simulink model "Ecotron"  (R2019b)
settings: Solver=FixedStepAuto  StartTime=0.0  StopTime=1  FixedStep=0.001  RelTol=1e-3  EnableMultiTasking=on
InitFcn:
  | EcoCoder_PreCheckLic();
libraries: CoderSF_BSW_Libs x228, SF_CanService_Libs x49, simulink x33, dspstat3 x6
(part 5 of 6)

== system Ecotron/Input/PC/FrontWheelCommands/Subsystem1 ==
  "Available_in " : Inport
  Msg_cnt : Inport  Port=2
  Constant : Constant  Value=3  OutDataTypeStr=single
  Data Type Conversion : DataTypeConversion  OutDataTypeStr=single
  Delay1 : Delay  InitialCondition=0  SampleTime=0.5
  Delay2 : Delay  DelayLength=6  InitialCondition=0  SampleTime=0.5
  Delay3 : Delay  DelayLength=0  InitialCondition=0  SampleTime=0.5
  Divide : Product  Inputs=*/
  Relational Operator : RelationalOperator  Operator===  OutDataTypeStr=boolean  RndMeth=Simplest
  Subtract : Sum  Inputs=+-
  Write Measurement : CoderSF_BSW_Libs/Calibration & Measurement/Write Measurement  variable_name=PC_FrontwheelMsg_cnt  variable_value=0  variable_type=uint32  numD=1  unitStr=""  descStr=""
      settings: AttributesFormatString=type:%<variable_type> Dimensions:%<numD>  SourceProductName=EcoCoder Blocks
  Write Measurement1 : CoderSF_BSW_Libs/Calibration & Measurement/Write Measurement  variable_name=PC_FrontwheelMsg_Freq  variable_value=0  variable_type=single  numD=1  unitStr=""  descStr=""
      settings: AttributesFormatString=type:%<variable_type> Dimensions:%<numD>  SourceProductName=EcoCoder Blocks
  "Available " : Outport
  Cnt : Outport  Port=2
  Timeout_Err : Outport  Port=3
  Msg_Freq : Outport  Port=4
  wires:
  Delay3/1 -> Subtract/1
  Constant/1 -> Divide/2
  Divide/1 -> Write Measurement1/1, Msg_Freq/1
  Data Type Conversion/1 -> Divide/1
  Delay2/1 -> Subtract/2
  Delay1/1 -> Relational Operator/2
  Msg_cnt/1 -> Cnt/1, Delay2/1, Delay1/1, Write Measurement/1, Relational Operator/1, Delay3/1
  Relational Operator/1 -> Timeout_Err/1
  Subtract/1 -> Data Type Conversion/1
  "Available_in "/1 -> "Available "/1

== system Ecotron/Input/PC/LongitudinalCommands/Subsystem1 ==
  "Available_in " : Inport
  Msg_cnt : Inport  Port=2
  Constant : Constant  Value=3  OutDataTypeStr=single
  Data Type Conversion : DataTypeConversion  OutDataTypeStr=single
  Delay1 : Delay  InitialCondition=0  SampleTime=0.5
  Delay2 : Delay  DelayLength=6  InitialCondition=0  SampleTime=0.5
  Delay3 : Delay  DelayLength=0  InitialCondition=0  SampleTime=0.5
  Divide : Product  Inputs=*/
  Relational Operator : RelationalOperator  Operator===  OutDataTypeStr=boolean  RndMeth=Simplest
  Subtract : Sum  Inputs=+-
  "Available " : Outport
  Cnt : Outport  Port=2
  Timeout_Err : Outport  Port=3
  Msg_Freq : Outport  Port=4
  wires:
  "Available_in "/1 -> "Available "/1
  Subtract/1 -> Data Type Conversion/1
  Relational Operator/1 -> Timeout_Err/1
  Msg_cnt/1 -> Relational Operator/1, Delay3/1, Delay1/1, Delay2/1, Cnt/1
  Delay1/1 -> Relational Operator/2
  Delay2/1 -> Subtract/2
  Data Type Conversion/1 -> Divide/1
  Divide/1 -> Msg_Freq/1
  Constant/1 -> Divide/2
  Delay3/1 -> Subtract/1

== system Ecotron/Input/PC/LongitudinalCommandsV2/Subsystem1 ==
  "Available_in " : Inport
  Msg_cnt : Inport  Port=2
  Constant : Constant  Value=3  OutDataTypeStr=single
  Data Type Conversion : DataTypeConversion  OutDataTypeStr=single
  Delay1 : Delay  InitialCondition=0  SampleTime=0.5
  Delay2 : Delay  DelayLength=6  InitialCondition=0  SampleTime=0.5
  Delay3 : Delay  DelayLength=0  InitialCondition=0  SampleTime=0.5
  Divide : Product  Inputs=*/
  Relational Operator : RelationalOperator  Operator===  OutDataTypeStr=boolean  RndMeth=Simplest
  Subtract : Sum  Inputs=+-
  "Available " : Outport
  Cnt : Outport  Port=2
  Timeout_Err : Outport  Port=3
  Msg_Freq : Outport  Port=4
  wires:
  Delay3/1 -> Subtract/1
  Constant/1 -> Divide/2
  Divide/1 -> Msg_Freq/1
  Data Type Conversion/1 -> Divide/1
  Delay2/1 -> Subtract/2
  Delay1/1 -> Relational Operator/2
  Msg_cnt/1 -> Cnt/1, Delay2/1, Delay1/1, Delay3/1, Relational Operator/1
  Relational Operator/1 -> Timeout_Err/1
  Subtract/1 -> Data Type Conversion/1
  "Available_in "/1 -> "Available "/1

== system Ecotron/Input/PC/Vehicle_Commands/Subsystem1 ==
  "Available_in " : Inport
  Msg_cnt : Inport  Port=2
  Constant : Constant  Value=3  OutDataTypeStr=single
  Data Type Conversion : DataTypeConversion  OutDataTypeStr=single
  Delay1 : Delay  InitialCondition=0  SampleTime=0.5
  Delay2 : Delay  DelayLength=6  InitialCondition=0  SampleTime=0.5
  Delay3 : Delay  DelayLength=0  InitialCondition=0  SampleTime=0.5
  Divide : Product  Inputs=*/
  Relational Operator : RelationalOperator  Operator===  OutDataTypeStr=boolean  RndMeth=Simplest
  Subtract : Sum  Inputs=+-
  "Available " : Outport
  Cnt : Outport  Port=2
  Timeout_Err : Outport  Port=3
  Msg_Freq : Outport  Port=4
  wires:
  Delay3/1 -> Subtract/1
  Constant/1 -> Divide/2
  Divide/1 -> Msg_Freq/1
  Data Type Conversion/1 -> Divide/1
  Delay2/1 -> Subtract/2
  Delay1/1 -> Relational Operator/2
  Msg_cnt/1 -> Cnt/1, Delay2/1, Delay1/1, Delay3/1, Relational Operator/1
  Relational Operator/1 -> Timeout_Err/1
  Subtract/1 -> Data Type Conversion/1
  "Available_in "/1 -> "Available "/1

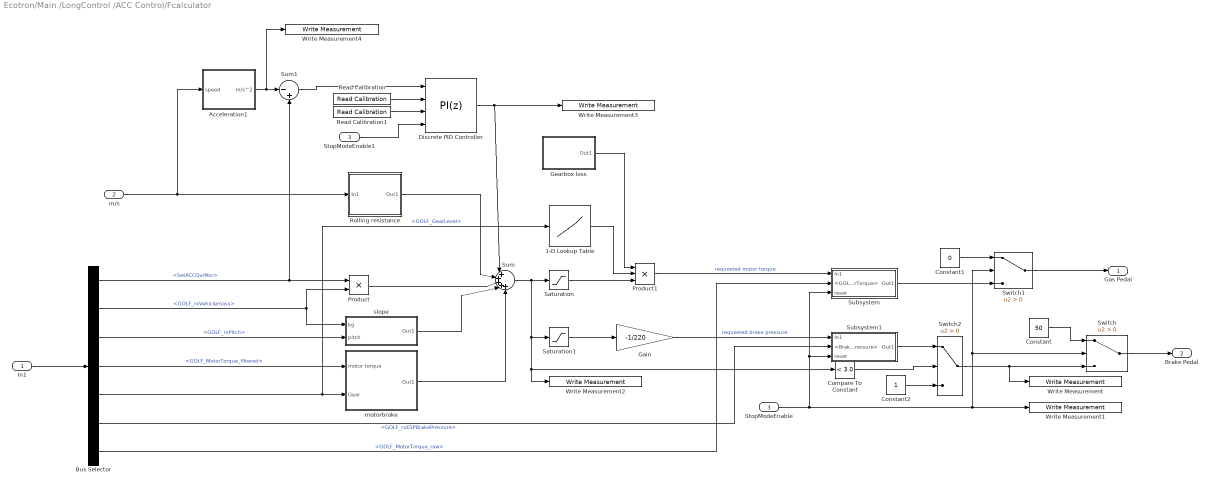
== system Ecotron/Main /LongControl /ACC Control/Fcalculator  ==
  In1 : Inport
  m/s : Inport  Port=2
  StopModeEnable : Inport  Port=3
  1-D Lookup Table : Lookup_n-D  NumberOfTableDimensions=1  BreakpointsForDimension1=[0 1 2 3 4 5]  Table=[0 1/53.5 1/32.6 1/21.7 1/16.2 1/12.2]  InternalRulePriority=Speed  RndMeth=Simplest  InputSameDT=on
  Acceleration1 : Subsystem
  Bus Selector : BusSelector  OutputSignals=input.PC.LongCMD.SetACCOvrMsr,input.vehicle.TSK.GOLF_rxVehiclemass,input.vehicle.TSK.GOLF_rxPitch,input.vehicle.MotorTorque.GOLF_MotorTorque_filtered,input.vehicle.GearLevel.GOLF_GearLevel,input.vehicle.BrakePressure.GOLF_rxESPBrakePressure,input.vehicle.MotorTorque.GOLF_MotorTorque_raw
  Compare To Constant : simulink/Logic and Bit Operations/Compare To Constant  relop=<  const=3.0  OutDataTypeStr=boolean
  Constant : Constant  Value=50  OutDataTypeStr=single
  Constant1 : Constant  Value=0  OutDataTypeStr=single
  Constant2 : Constant
  Discrete PID Controller : simulink/Continuous/PID Controller  Controller=PI  Form=Parallel  TimeDomain=Discrete-time  SampleTime=-1  IntegratorMethod=Forward Euler  FilterMethod=Forward Euler  ControllerParametersSource=external  P=1  I=1  D=0  UseFilter=off  N=100  TunerSelectOption=Transfer Function Based (PID Tuner App)  InitialConditionSource=internal  InitialConditionForIntegrator=0  InitialConditionForFilter=0  DifferentiatorICPrevScaledInput=0  ExternalReset=either  TrackingMode=off  Kt=1  LimitOutput=on  UpperSaturationLimit=300  LowerSaturationLimit=-300  LinearizeAsGain=off  AntiWindupMode=clamping  Kb=1  POutMin=[]  POutMax=[]  IOutMin=[]  IOutMax=[]  DOutMin=[]  DOutMax=[]  NOutMin=[]  NOutMax=[]  SumOutMin=[]  SumOutMax=[]  SaturationOutMin=[]  SaturationOutMax=[]  PParamMin=[]  PParamMax=[]  IParamMin=[]  IParamMax=[]  DParamMin=[]  DParamMax=[]  NParamMin=[]  NParamMax=[]  KbParamMin=[]  KbParamMax=[]  KtParamMin=[]  KtParamMax=[]  KbOutMin=[]  KbOutMax=[]  KtOutMin=[]  KtOutMax=[]  IntegratorOutMin=[]  IntegratorOutMax=[]  FilterOutMin=[]  FilterOutMax=[]  SumI1OutMin=[]  SumI1OutMax=[]  SumI2OutMin=[]  SumI2OutMax=[]  SumI3OutMin=[]  SumI3OutMax=[]  SumI4OutMin=[]  SumI4OutMax=[]  SumDOutMin=[]  SumDOutMax=[]  DifferentiatorOutMin=[]  DifferentiatorOutMax=[]  FilterDiffOutCoefMin=[]  FilterDiffOutCoefMax=[]  ReciprocalOutMin=[]  ReciprocalOutMax=[]  SumDenOutMin=[]  SumDenOutMax=[]  SumNumOutMin=[]  SumNumOutMax=[]  DivideOutMin=[]  DivideOutMax=[]  IntegratorContinuousStateAttributes=''  IntegratorStateMustResolveToSignalObject=off  IntegratorRTWStateStorageClass=Auto  FilterContinuousStateAttributes=''  FilterStateMustResolveToSignalObject=off  FilterRTWStateStorageClass=Auto  ParallelPVariant=ExternalParameters  IdealPVariant=Disabled  IVariant=ExternalParameters  DVariant=Disabled  IntegratorVariant=Discrete  SatVariant=Enabled  AWVariant=DiscClampingParallel  PCopyVariant=Disabled  TRVariant=Disabled  FdbkBlocksVariant=Forward  IdealPFdbkVariant=Disabled  SatFdbkVariant=Disabled  DerivativeFilterVariant=Disabled  NVariant=Disabled  NCopyVariant=Disabled_SignalSpec  FilterICVariant=Disabled  IntegratorICVariant=InternalICs  ExternalResetVariant=ExternalReset  TRSumVariant=Passthrough  SumFdbkVariant=Disabled  SumVariant=Sum_PI
  Gain : Gain  Gain=-1/220
  Gearbox loss : Subsystem
  Product : Product
  Product1 : Product  Inputs=3
  Read Calibration : CoderSF_BSW_Libs/Calibration & Measurement/Read Calibration  variable_name=Compensation_P  variable_value=300  variable_type=single  variable_min=[]  variable_max=[]  unitStr=""  descStr=""
      settings: AttributesFormatString=value:%<variable_value> type:%<variable_type> max:%<variable_max> Min:%<variable_min>
  Read Calibration1 : CoderSF_BSW_Libs/Calibration & Measurement/Read Calibration  variable_name=Compensation_I  variable_value=300  variable_type=single  variable_min=[]  variable_max=[]  unitStr=""  descStr=""
      settings: AttributesFormatString=value:%<variable_value> type:%<variable_type> max:%<variable_max> Min:%<variable_min>
  Rolling resistance : Subsystem
  Saturation : Saturate  UpperLimit=3000  LowerLimit=0
  Saturation1 : Saturate  UpperLimit=10  LowerLimit=-10000
  StopModeEnable1 : InportShadow  Port=3
  Subsystem : Subsystem
  Subsystem1 : Subsystem
  Sum : Sum  Inputs=|+++++
  Sum1 : Sum  Inputs=|-+
  Switch : Switch  Criteria=u2 > Threshold
  Switch1 : Switch  Criteria=u2 > Threshold
  Switch2 : Switch  Criteria=u2 > Threshold
  Write Measurement : CoderSF_BSW_Libs/Calibration & Measurement/Write Measurement  variable_name=debug_set_brake  variable_value=0  variable_type=single  numD=1  unitStr=""  descStr=""
      settings: AttributesFormatString=type:%<variable_type> Dimensions:%<numD>
  Write Measurement1 : CoderSF_BSW_Libs/Calibration & Measurement/Write Measurement  variable_name=debug_stopmode  variable_value=0  variable_type=boolean  numD=1  unitStr=""  descStr=""
      settings: AttributesFormatString=type:%<variable_type> Dimensions:%<numD>
  Write Measurement2 : CoderSF_BSW_Libs/Calibration & Measurement/Write Measurement  variable_name=debug_Fr_request  variable_value=0  variable_type=single  numD=1  unitStr=""  descStr=""
      settings: AttributesFormatString=type:%<variable_type> Dimensions:%<numD>
  Write Measurement3 : CoderSF_BSW_Libs/Calibration & Measurement/Write Measurement  variable_name=debug_CompensationPID_out  variable_value=0  variable_type=single  numD=1  unitStr=""  descStr=""
      settings: AttributesFormatString=type:%<variable_type> Dimensions:%<numD>
  Write Measurement4 : CoderSF_BSW_Libs/Calibration & Measurement/Write Measurement  variable_name=debug_filtered_ACC  variable_value=0  variable_type=single  numD=1  unitStr=""  descStr=""
      settings: AttributesFormatString=type:%<variable_type> Dimensions:%<numD>
  motorbrake : Subsystem
  slope : Subsystem
  Gas Pedal : Outport
  Brake Pedal : Outport  Port=2
  wires:
  In1/1 -> Bus Selector/1
  m/s/1 -> Acceleration1/1(speed), Rolling resistance/1(In1)
  Bus Selector/3 -> slope/2(pitch)  "<GOLF_rxPitch>"
  Bus Selector/2 -> slope/1(kg), Product/2  "<GOLF_rxVehiclemass>"
  Bus Selector/1 -> Sum1/2, Product/1  "<SetACCOvrMsr>"
  Bus Selector/4 -> motorbrake/1(motor torque)  "<GOLF_MotorTorque_filtered>"
  Bus Selector/5 -> motorbrake/2(Gear), 1-D Lookup Table/1  "<GOLF_GearLevel>"
  Rolling resistance/1(Out1) -> Sum/2
  Product/1 -> Sum/3
  slope/1(Out1) -> Sum/4
  motorbrake/1(Out1) -> Sum/5
  Sum/1 -> Write Measurement2/1, Compare To Constant/1, Saturation1/1, Saturation/1
  1-D Lookup Table/1 -> Product1/2
  Saturation/1 -> Product1/3
  Gearbox loss/1(Out1) -> Product1/1
  Saturation1/1 -> Gain/1
  Product1/1 -> Subsystem/1(In1)  "requested motor torque"
  Gain/1 -> Subsystem1/1(In1)  "requested brake pressure"
  Bus Selector/6 -> Subsystem1/2(<Brake pressure>)  "<GOLF_rxESPBrakePressure>"
  Constant1/1 -> Switch1/1
  Constant/1 -> Switch/1
  Subsystem/1(Out1) -> Switch1/3
  Switch1/1 -> Gas Pedal/1
  Switch2/1 -> Write Measurement/1, Switch/3
  Switch/1 -> Brake Pedal/1
  StopModeEnable/1 -> Subsystem/3(reset), Subsystem1/3(reset), Switch1/2, Switch/2, Write Measurement1/1
  Acceleration1/1(m/s^2) -> Write Measurement4/1, Sum1/1
  Sum1/1 -> Discrete PID Controller/1
  StopModeEnable1/1 -> Discrete PID Controller/4
  Read Calibration/1 -> Discrete PID Controller/2
  Read Calibration1/1 -> Discrete PID Controller/3
  Discrete PID Controller/1 -> Write Measurement3/1, Sum/1
  Bus Selector/7 -> Subsystem/2(<GOLF_MotorTorque>)  "<GOLF_MotorTorque_raw>"
  Subsystem1/1(Out1) -> Switch2/1
  Compare To Constant/1 -> Switch2/2
  Constant2/1 -> Switch2/3

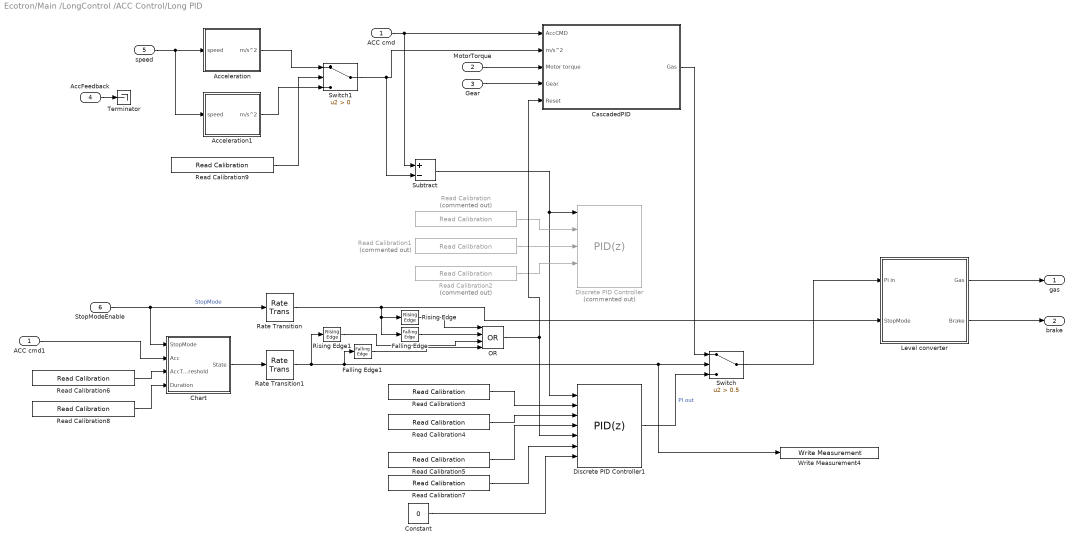
== system Ecotron/Main /LongControl /ACC Control/Long PID ==
  ACC cmd : Inport
  MotorTorque : Inport  Port=2
  Gear : Inport  Port=3
  AccFeedback : Inport  Port=4
  speed : Inport  Port=5
  StopModeEnable : Inport  Port=6
  ACC cmd1 : InportShadow
  Acceleration : Subsystem
  Acceleration1 : Subsystem
  CascadedPID : Subsystem
  Chart : Stateflow chart  BlockKeywords=__PRM__SERIALIZED__DATA__:Stateflow Chart,Stateflow Diagram  TreatAsAtomicUnit=on
  Constant : Constant  Value=0  OutDataTypeStr=single
  Discrete PID Controller : simulink/Continuous/PID Controller  Commented=on  Controller=PID  Form=Parallel  TimeDomain=Discrete-time  SampleTime=1/100  IntegratorMethod=Forward Euler  FilterMethod=Forward Euler  ControllerParametersSource=external  P=1  I=1  D=0  UseFilter=off  N=100  TunerSelectOption=Transfer Function Based (PID Tuner App)  ZeroCross=off  InitialConditionSource=internal  InitialConditionForIntegrator=0  InitialConditionForFilter=0  DifferentiatorICPrevScaledInput=0  ExternalReset=either  TrackingMode=off  Kt=1  LimitOutput=on  UpperSaturationLimit=0.5  LowerSaturationLimit=-0.1  LinearizeAsGain=off  AntiWindupMode=clamping  Kb=1  POutMin=[]  POutMax=[]  IOutMin=[]  IOutMax=[]  DOutMin=[]  DOutMax=[]  NOutMin=[]  NOutMax=[]  SumOutMin=[]  SumOutMax=[]  SaturationOutMin=[]  SaturationOutMax=[]  PParamMin=[]  PParamMax=[]  IParamMin=[]  IParamMax=[]  DParamMin=[]  DParamMax=[]  NParamMin=[]  NParamMax=[]  KbParamMin=[]  KbParamMax=[]  KtParamMin=[]  KtParamMax=[]  KbOutMin=[]  KbOutMax=[]  KtOutMin=[]  KtOutMax=[]  IntegratorOutMin=[]  IntegratorOutMax=[]  FilterOutMin=[]  FilterOutMax=[]  SumI1OutMin=[]  SumI1OutMax=[]  SumI2OutMin=[]  SumI2OutMax=[]  SumI3OutMin=[]  SumI3OutMax=[]  SumI4OutMin=[]  SumI4OutMax=[]  SumDOutMin=[]  SumDOutMax=[]  DifferentiatorOutMin=[]  DifferentiatorOutMax=[]  FilterDiffOutCoefMin=[]  FilterDiffOutCoefMax=[]  ReciprocalOutMin=[]  ReciprocalOutMax=[]  SumDenOutMin=[]  SumDenOutMax=[]  SumNumOutMin=[]  SumNumOutMax=[]  DivideOutMin=[]  DivideOutMax=[]  IntegratorContinuousStateAttributes=''  IntegratorStateMustResolveToSignalObject=off  IntegratorRTWStateStorageClass=Auto  FilterContinuousStateAttributes=''  FilterStateMustResolveToSignalObject=off  FilterRTWStateStorageClass=Auto  ParallelPVariant=ExternalParameters  IdealPVariant=Disabled  IVariant=ExternalParameters  DVariant=ExternalParameters  IntegratorVariant=Discrete  SatVariant=Enabled  AWVariant=DiscClampingParallel  PCopyVariant=Disabled  TRVariant=Disabled  FdbkBlocksVariant=Forward  IdealPFdbkVariant=Disabled  SatFdbkVariant=Disabled  DerivativeFilterVariant=Differentiator  NVariant=Passthrough  NCopyVariant=Disabled_SignalSpec  FilterICVariant=InternalICsDifferentiator  IntegratorICVariant=InternalICs  ExternalResetVariant=ExternalReset  TRSumVariant=Passthrough  SumFdbkVariant=Disabled  SumVariant=Sum_PID
  Discrete PID Controller1 : simulink/Continuous/PID Controller  Controller=PID  Form=Parallel  TimeDomain=Discrete-time  SampleTime=1/100  IntegratorMethod=Forward Euler  FilterMethod=Forward Euler  ControllerParametersSource=external  P=1  I=1  D=0  UseFilter=off  N=100  TunerSelectOption=Transfer Function Based (PID Tuner App)  ZeroCross=off  InitialConditionSource=external  InitialConditionForIntegrator=0  InitialConditionForFilter=0  DifferentiatorICPrevScaledInput=0  ExternalReset=either  TrackingMode=off  Kt=1  LimitOutput=on  UpperSaturationLimit=0.05  LowerSaturationLimit=-1  LinearizeAsGain=off  AntiWindupMode=clamping  Kb=1  POutMin=[]  POutMax=[]  IOutMin=[]  IOutMax=[]  DOutMin=[]  DOutMax=[]  NOutMin=[]  NOutMax=[]  SumOutMin=[]  SumOutMax=[]  SaturationOutMin=[]  SaturationOutMax=[]  PParamMin=[]  PParamMax=[]  IParamMin=[]  IParamMax=[]  DParamMin=[]  DParamMax=[]  NParamMin=[]  NParamMax=[]  KbParamMin=[]  KbParamMax=[]  KtParamMin=[]  KtParamMax=[]  KbOutMin=[]  KbOutMax=[]  KtOutMin=[]  KtOutMax=[]  IntegratorOutMin=[]  IntegratorOutMax=[]  FilterOutMin=[]  FilterOutMax=[]  SumI1OutMin=[]  SumI1OutMax=[]  SumI2OutMin=[]  SumI2OutMax=[]  SumI3OutMin=[]  SumI3OutMax=[]  SumI4OutMin=[]  SumI4OutMax=[]  SumDOutMin=[]  SumDOutMax=[]  DifferentiatorOutMin=[]  DifferentiatorOutMax=[]  FilterDiffOutCoefMin=[]  FilterDiffOutCoefMax=[]  ReciprocalOutMin=[]  ReciprocalOutMax=[]  SumDenOutMin=[]  SumDenOutMax=[]  SumNumOutMin=[]  SumNumOutMax=[]  DivideOutMin=[]  DivideOutMax=[]  IntegratorContinuousStateAttributes=''  IntegratorStateMustResolveToSignalObject=off  IntegratorRTWStateStorageClass=Auto  FilterContinuousStateAttributes=''  FilterStateMustResolveToSignalObject=off  FilterRTWStateStorageClass=Auto  ParallelPVariant=ExternalParameters  IdealPVariant=Disabled  IVariant=ExternalParameters  DVariant=ExternalParameters  IntegratorVariant=Discrete  SatVariant=Enabled  AWVariant=DiscClampingParallel  PCopyVariant=Disabled  TRVariant=Disabled  FdbkBlocksVariant=Forward  IdealPFdbkVariant=Disabled  SatFdbkVariant=Disabled  DerivativeFilterVariant=Differentiator  NVariant=Passthrough  NCopyVariant=Disabled_SignalSpec  FilterICVariant=ExternalICs  IntegratorICVariant=ExternalICs  ExternalResetVariant=ExternalReset  TRSumVariant=Passthrough  SumFdbkVariant=Disabled  SumVariant=Sum_PID
  Falling Edge : CoderSF_BSW_Libs/Application Base Blocks/Falling Edge  InitialCondition=off
      settings: SourceProductName=EcoCoder Blocks
  Falling Edge1 : CoderSF_BSW_Libs/Application Base Blocks/Falling Edge  InitialCondition=off
      settings: SourceProductName=EcoCoder Blocks
  Level converter : Subsystem
  OR : Logic  Operator=OR  Inputs=4  IconShape=distinctive  AllPortsSameDT=off  OutDataTypeStr=boolean
  Rate Transition : RateTransition  OutPortSampleTime=0.01
  Rate Transition1 : RateTransition  OutPortSampleTime=0.01
  Read Calibration : CoderSF_BSW_Libs/Calibration & Measurement/Read Calibration  Commented=on  variable_name=Acc_PID_P  variable_value=0.08  variable_type=single  variable_min=[]  variable_max=[]  unitStr=""  descStr=""
      settings: AttributesFormatString=value:%<variable_value> type:%<variable_type> max:%<variable_max> Min:%<variable_min>  SourceProductName=EcoCoder Blocks
  Read Calibration1 : CoderSF_BSW_Libs/Calibration & Measurement/Read Calibration  Commented=on  variable_name=Acc_PID_I  variable_value=0.15  variable_type=single  variable_min=[]  variable_max=[]  unitStr=""  descStr=""
      settings: AttributesFormatString=value:%<variable_value> type:%<variable_type> max:%<variable_max> Min:%<variable_min>  SourceProductName=EcoCoder Blocks
  Read Calibration2 : CoderSF_BSW_Libs/Calibration & Measurement/Read Calibration  Commented=on  variable_name=Acc_PID_D  variable_value=0.0  variable_type=single  variable_min=[]  variable_max=[]  unitStr=""  descStr=""
      settings: AttributesFormatString=value:%<variable_value> type:%<variable_type> max:%<variable_max> Min:%<variable_min>  SourceProductName=EcoCoder Blocks
  Read Calibration3 : CoderSF_BSW_Libs/Calibration & Measurement/Read Calibration  variable_name=Decc_PID_P  variable_value=0.05  variable_type=single  variable_min=[]  variable_max=[]  unitStr=""  descStr=""
      settings: AttributesFormatString=value:%<variable_value> type:%<variable_type> max:%<variable_max> Min:%<variable_min>  SourceProductName=EcoCoder Blocks
  Read Calibration4 : CoderSF_BSW_Libs/Calibration & Measurement/Read Calibration  variable_name=Decc_PID_I  variable_value=0.35  variable_type=single  variable_min=[]  variable_max=[]  unitStr=""  descStr=""
      settings: AttributesFormatString=value:%<variable_value> type:%<variable_type> max:%<variable_max> Min:%<variable_min>  SourceProductName=EcoCoder Blocks
  Read Calibration5 : CoderSF_BSW_Libs/Calibration & Measurement/Read Calibration  variable_name=Decc_PID_D  variable_value=0.0  variable_type=single  variable_min=[]  variable_max=[]  unitStr=""  descStr=""
      settings: AttributesFormatString=value:%<variable_value> type:%<variable_type> max:%<variable_max> Min:%<variable_min>  SourceProductName=EcoCoder Blocks
  Read Calibration6 : CoderSF_BSW_Libs/Calibration & Measurement/Read Calibration  variable_name=Acc_Threshold  variable_value=0.08  variable_type=single  variable_min=[]  variable_max=[]  unitStr=""  descStr=""
      settings: AttributesFormatString=value:%<variable_value> type:%<variable_type> max:%<variable_max> Min:%<variable_min>  SourceProductName=EcoCoder Blocks
  Read Calibration7 : CoderSF_BSW_Libs/Calibration & Measurement/Read Calibration  variable_name=Decc_PID_I0  variable_value=-0.05  variable_type=single  variable_min=[]  variable_max=[]  unitStr=""  descStr=""
      settings: AttributesFormatString=value:%<variable_value> type:%<variable_type> max:%<variable_max> Min:%<variable_min>  SourceProductName=EcoCoder Blocks
  Read Calibration8 : CoderSF_BSW_Libs/Calibration & Measurement/Read Calibration  variable_name=Acc_Duration  variable_value=0.8  variable_type=single  variable_min=[]  variable_max=[]  unitStr=""  descStr=""
      settings: AttributesFormatString=value:%<variable_value> type:%<variable_type> max:%<variable_max> Min:%<variable_min>  SourceProductName=EcoCoder Blocks
  Read Calibration9 : CoderSF_BSW_Libs/Calibration & Measurement/Read Calibration  variable_name=ACC_feedback  variable_value=0  variable_type=boolean  variable_min=[]  variable_max=[]  unitStr=bool  descStr="0 -> speed Derivative  1-> CAN"
      settings: AttributesFormatString=value:%<variable_value> type:%<variable_type> max:%<variable_max> Min:%<variable_min>  SourceProductName=EcoCoder Blocks
  Rising Edge : CoderSF_BSW_Libs/Application Base Blocks/Rising Edge  InitialCondition=on
      settings: SourceProductName=EcoCoder Blocks
  Rising Edge1 : CoderSF_BSW_Libs/Application Base Blocks/Rising Edge  InitialCondition=on
      settings: SourceProductName=EcoCoder Blocks
  Subtract : Sum  Inputs=+-
  Switch : Switch  Criteria=u2 > Threshold  Threshold=0.5
  Switch1 : Switch  Criteria=u2 > Threshold
  Terminator : Terminator
  Write Measurement4 : CoderSF_BSW_Libs/Calibration & Measurement/Write Measurement  variable_name=GasBrakeMode  variable_value=0  variable_type=boolean  numD=1  unitStr=""  descStr=""
      settings: AttributesFormatString=type:%<variable_type> Dimensions:%<numD>  SourceProductName=EcoCoder Blocks
  gas : Outport
  brake : Outport  Port=2
  wires:
  ACC cmd/1 -> CascadedPID/1(AccCMD), Subtract/1
  Subtract/1 -> Discrete PID Controller1/1, Discrete PID Controller/1
  Read Calibration/1 -> Discrete PID Controller/2
  Read Calibration1/1 -> Discrete PID Controller/3
  StopModeEnable/1 -> Chart/1(StopMode), Rate Transition/1  "StopMode"
  Level converter/2(Brake) -> brake/1
  Level converter/1(Gas) -> gas/1
  Read Calibration2/1 -> Discrete PID Controller/4
  Read Calibration3/1 -> Discrete PID Controller1/2
  Read Calibration4/1 -> Discrete PID Controller1/3
  Read Calibration5/1 -> Discrete PID Controller1/4
  Read Calibration6/1 -> Chart/3(AccThreshold)
  Chart/1(State) -> Rate Transition1/1
  Discrete PID Controller1/1 -> Switch/3  "PI out"
  Switch/1 -> Level converter/1(Pi in)
  OR/1 -> CascadedPID/5("Reset "), Discrete PID Controller1/5
  Constant/1 -> Discrete PID Controller1/7
  Read Calibration7/1 -> Discrete PID Controller1/6
  Rising Edge/1 -> OR/1
  Falling Edge/1 -> OR/2
  Rising Edge1/1 -> OR/3
  Falling Edge1/1 -> OR/4
  Rate Transition/1 -> Falling Edge/1, Rising Edge/1, Level converter/2(StopMode)
  Rate Transition1/1 -> Falling Edge1/1, Write Measurement4/1, Switch/2, Rising Edge1/1
  speed/1 -> Acceleration1/1(speed), Acceleration/1(speed)
  MotorTorque/1 -> CascadedPID/3(Motor torque)
  Gear/1 -> CascadedPID/4(Gear)
  CascadedPID/1(Gas) -> Switch/1
  Read Calibration8/1 -> Chart/4(Duration)
  Acceleration/1(m/s^2) -> Switch1/1
  Switch1/1 -> Subtract/2, CascadedPID/2(m/s^2)
  Read Calibration9/1 -> Switch1/2
  AccFeedback/1 -> Terminator/1
  Acceleration1/1(m/s^2) -> Switch1/3
  ACC cmd1/1 -> Chart/2(Acc)

== system Ecotron/Main /LongControl /ACC Control/StopModeDesicion ==
  note: 1 P
      | 2 R
      | 3 N
      | 4 D
  speed : Inport
  bus : Inport  Port=2
  Bus Selector : BusSelector  OutputSignals=input.PC.LongCMD.SetACCOvrMsr,input.vehicle.gear.GOLF_CurrentGear,mode
  Chart1 : Stateflow chart  BlockKeywords=__PRM__SERIALIZED__DATA__:Stateflow Chart,Stateflow Diagram  TreatAsAtomicUnit=on
  StopModeEnable : Outport
  wires:
  bus/1 -> Bus Selector/1
  speed/1 -> Chart1/4(Speed)
  Bus Selector/2 -> Chart1/2(Gear)  "<GOLF_CurrentGear>"
  Bus Selector/1 -> Chart1/1(Acc)  "<SetACCOvrMsr>"
  Chart1/1(Stopmode) -> StopModeEnable/1
  Bus Selector/3 -> Chart1/3(mode)  "<mode>"

== system Ecotron/Main /LongControl /ACC Control/VehicleSpeed ==
  In1 : Inport
  Bus Selector : BusSelector  OutputSignals=input.vehicle.WheelSpeed.GOLF_BLWheelSpeed,input.vehicle.WheelSpeed.GOLF_BRWheelSpeed
  Multiply : Gain  Gain=0.5
  Multiply1 : Gain  Gain=1/3.6
  Sum : Sum  Inputs=|++
  m/s : Outport
  wires:
  In1/1 -> Bus Selector/1
  Bus Selector/1 -> Sum/1  "<GOLF_BLWheelSpeed>"
  Bus Selector/2 -> Sum/2  "<GOLF_BRWheelSpeed>"
  Sum/1 -> Multiply/1
  Multiply/1 -> Multiply1/1
  Multiply1/1 -> m/s/1

== system Ecotron/Input/By-wire/PDS/Subsystem/Subsystem4 ==
  "Available_in " : Inport
  Msg_cnt : Inport  Port=2
  Constant : Constant  Value=3  OutDataTypeStr=single
  Data Type Conversion : DataTypeConversion  OutDataTypeStr=single
  Delay1 : Delay  InitialCondition=0  SampleTime=0.5
  Delay2 : Delay  DelayLength=6  InitialCondition=0  SampleTime=0.5
  Delay3 : Delay  DelayLength=0  InitialCondition=0  SampleTime=0.5
  Divide : Product  Inputs=*/
  Relational Operator : RelationalOperator  Operator===  OutDataTypeStr=boolean  RndMeth=Simplest
  Subtract : Sum  Inputs=+-
  "Available " : Outport
  Cnt : Outport  Port=2
  Timeout_Err : Outport  Port=3
  Msg_Freq : Outport  Port=4
  wires:
  "Available_in "/1 -> "Available "/1
  Subtract/1 -> Data Type Conversion/1
  Relational Operator/1 -> Timeout_Err/1
  Msg_cnt/1 -> Relational Operator/1, Delay3/1, Delay1/1, Delay2/1, Cnt/1
  Delay1/1 -> Relational Operator/2
  Delay2/1 -> Subtract/2
  Data Type Conversion/1 -> Divide/1
  Divide/1 -> Msg_Freq/1
  Constant/1 -> Divide/2
  Delay3/1 -> Subtract/1

== system Ecotron/Input/By-wire/PDS/Subsystem1/Subsystem6 ==
  "Available_in " : Inport
  Msg_cnt : Inport  Port=2
  Constant : Constant  Value=3  OutDataTypeStr=single
  Data Type Conversion : DataTypeConversion  OutDataTypeStr=single
  Delay1 : Delay  InitialCondition=0  SampleTime=0.5
  Delay2 : Delay  DelayLength=6  InitialCondition=0  SampleTime=0.5
  Delay3 : Delay  DelayLength=0  InitialCondition=0  SampleTime=0.5
  Divide : Product  Inputs=*/
  Relational Operator : RelationalOperator  Operator===  OutDataTypeStr=boolean  RndMeth=Simplest
  Subtract : Sum  Inputs=+-
  "Available " : Outport
  Cnt : Outport  Port=2
  Timeout_Err : Outport  Port=3
  Msg_Freq : Outport  Port=4
  wires:
  "Available_in "/1 -> "Available "/1
  Subtract/1 -> Data Type Conversion/1
  Relational Operator/1 -> Timeout_Err/1
  Msg_cnt/1 -> Relational Operator/1, Delay3/1, Delay1/1, Delay2/1, Cnt/1
  Delay1/1 -> Relational Operator/2
  Delay2/1 -> Subtract/2
  Data Type Conversion/1 -> Divide/1
  Divide/1 -> Msg_Freq/1
  Constant/1 -> Divide/2
  Delay3/1 -> Subtract/1

== system Ecotron/Input/By-wire/PDS/Subsystem2/Subsystem1 ==
  "Available_in " : Inport
  Msg_cnt : Inport  Port=2
  Constant : Constant  Value=3  OutDataTypeStr=single
  Data Type Conversion : DataTypeConversion  OutDataTypeStr=single
  Delay1 : Delay  InitialCondition=0  SampleTime=0.5
  Delay2 : Delay  DelayLength=6  InitialCondition=0  SampleTime=0.5
  Delay3 : Delay  DelayLength=0  InitialCondition=0  SampleTime=0.5
  Divide : Product  Inputs=*/
  Relational Operator : RelationalOperator  Operator===  OutDataTypeStr=boolean  RndMeth=Simplest
  Subtract : Sum  Inputs=+-
  "Available " : Outport
  Cnt : Outport  Port=2
  Timeout_Err : Outport  Port=3
  Msg_Freq : Outport  Port=4
  wires:
  "Available_in "/1 -> "Available "/1
  Subtract/1 -> Data Type Conversion/1
  Relational Operator/1 -> Timeout_Err/1
  Msg_cnt/1 -> Relational Operator/1, Delay3/1, Delay1/1, Delay2/1, Cnt/1
  Delay1/1 -> Relational Operator/2
  Delay2/1 -> Subtract/2
  Data Type Conversion/1 -> Divide/1
  Divide/1 -> Msg_Freq/1
  Constant/1 -> Divide/2
  Delay3/1 -> Subtract/1

== system Ecotron/Input/By-wire/PDS/Subsystem3/Subsystem2 ==
  "Available_in " : Inport
  Msg_cnt : Inport  Port=2
  Constant : Constant  Value=3  OutDataTypeStr=single
  Data Type Conversion : DataTypeConversion  OutDataTypeStr=single
  Delay1 : Delay  InitialCondition=0  SampleTime=0.5
  Delay2 : Delay  DelayLength=6  InitialCondition=0  SampleTime=0.5
  Delay3 : Delay  DelayLength=0  InitialCondition=0  SampleTime=0.5
  Divide : Product  Inputs=*/
  Relational Operator : RelationalOperator  Operator===  OutDataTypeStr=boolean  RndMeth=Simplest
  Subtract : Sum  Inputs=+-
  "Available " : Outport
  Cnt : Outport  Port=2
  Timeout_Err : Outport  Port=3
  Msg_Freq : Outport  Port=4
  wires:
  "Available_in "/1 -> "Available "/1
  Subtract/1 -> Data Type Conversion/1
  Relational Operator/1 -> Timeout_Err/1
  Msg_cnt/1 -> Relational Operator/1, Delay3/1, Delay1/1, Delay2/1, Cnt/1
  Delay1/1 -> Relational Operator/2
  Delay2/1 -> Subtract/2
  Data Type Conversion/1 -> Divide/1
  Divide/1 -> Msg_Freq/1
  Constant/1 -> Divide/2
  Delay3/1 -> Subtract/1

== system Ecotron/Input/By-wire/PDS/Subsystem4/Subsystem3 ==
  "Available_in " : Inport
  Msg_cnt : Inport  Port=2
  Constant : Constant  Value=3  OutDataTypeStr=single
  Data Type Conversion : DataTypeConversion  OutDataTypeStr=single
  Delay1 : Delay  InitialCondition=0  SampleTime=0.5
  Delay2 : Delay  DelayLength=6  InitialCondition=0  SampleTime=0.5
  Delay3 : Delay  DelayLength=0  InitialCondition=0  SampleTime=0.5
  Divide : Product  Inputs=*/
  Relational Operator : RelationalOperator  Operator===  OutDataTypeStr=boolean  RndMeth=Simplest
  Subtract : Sum  Inputs=+-
  "Available " : Outport
  Cnt : Outport  Port=2
  Timeout_Err : Outport  Port=3
  Msg_Freq : Outport  Port=4
  wires:
  "Available_in "/1 -> "Available "/1
  Subtract/1 -> Data Type Conversion/1
  Relational Operator/1 -> Timeout_Err/1
  Msg_cnt/1 -> Relational Operator/1, Delay3/1, Delay1/1, Delay2/1, Cnt/1
  Delay1/1 -> Relational Operator/2
  Delay2/1 -> Subtract/2
  Data Type Conversion/1 -> Divide/1
  Divide/1 -> Msg_Freq/1
  Constant/1 -> Divide/2
  Delay3/1 -> Subtract/1

== system Ecotron/Input/By-wire/PDS/Subsystem6/Subsystem5 ==
  "Available_in " : Inport
  Msg_cnt : Inport  Port=2
  Constant : Constant  Value=3  OutDataTypeStr=single
  Data Type Conversion : DataTypeConversion  OutDataTypeStr=single
  Delay1 : Delay  InitialCondition=0  SampleTime=0.5
  Delay2 : Delay  DelayLength=6  InitialCondition=0  SampleTime=0.5
  Delay3 : Delay  DelayLength=0  InitialCondition=0  SampleTime=0.5
  Divide : Product  Inputs=*/
  Relational Operator : RelationalOperator  Operator===  OutDataTypeStr=boolean  RndMeth=Simplest
  Subtract : Sum  Inputs=+-
  "Available " : Outport
  Cnt : Outport  Port=2
  Timeout_Err : Outport  Port=3
  Msg_Freq : Outport  Port=4
  wires:
  "Available_in "/1 -> "Available "/1
  Subtract/1 -> Data Type Conversion/1
  Relational Operator/1 -> Timeout_Err/1
  Msg_cnt/1 -> Relational Operator/1, Delay3/1, Delay1/1, Delay2/1, Cnt/1
  Delay1/1 -> Relational Operator/2
  Delay2/1 -> Subtract/2
  Data Type Conversion/1 -> Divide/1
  Divide/1 -> Msg_Freq/1
  Constant/1 -> Divide/2
  Delay3/1 -> Subtract/1

== system Ecotron/Input/By-wire/Robeff Brake ECU/Robeff Brake FbMsg1/Subsystem4 ==
  "Available_in " : Inport
  Msg_cnt : Inport  Port=2
  Constant : Constant  Value=3  OutDataTypeStr=single
  Data Type Conversion : DataTypeConversion  OutDataTypeStr=single
  Delay1 : Delay  InitialCondition=0  SampleTime=0.5
  Delay2 : Delay  DelayLength=6  InitialCondition=0  SampleTime=0.5
  Delay3 : Delay  DelayLength=0  InitialCondition=0  SampleTime=0.5
  Divide : Product  Inputs=*/
  Relational Operator : RelationalOperator  Operator===  OutDataTypeStr=boolean  RndMeth=Simplest
  Subtract : Sum  Inputs=+-
  "Available " : Outport
  Cnt : Outport  Port=2
  Timeout_Err : Outport  Port=3
  Msg_Freq : Outport  Port=4
  wires:
  Delay3/1 -> Subtract/1
  Constant/1 -> Divide/2
  Divide/1 -> Msg_Freq/1
  Data Type Conversion/1 -> Divide/1
  Delay2/1 -> Subtract/2
  Delay1/1 -> Relational Operator/2
  Msg_cnt/1 -> Cnt/1, Delay2/1, Delay1/1, Delay3/1, Relational Operator/1
  Relational Operator/1 -> Timeout_Err/1
  Subtract/1 -> Data Type Conversion/1
  "Available_in "/1 -> "Available "/1

== system Ecotron/Input/By-wire/Robeff Brake ECU/Robeff Brake FbMsg2/Subsystem4 ==
  "Available_in " : Inport
  Msg_cnt : Inport  Port=2
  Constant : Constant  Value=3  OutDataTypeStr=single
  Data Type Conversion : DataTypeConversion  OutDataTypeStr=single
  Delay1 : Delay  InitialCondition=0  SampleTime=0.5
  Delay2 : Delay  DelayLength=6  InitialCondition=0  SampleTime=0.5
  Delay3 : Delay  DelayLength=0  InitialCondition=0  SampleTime=0.5
  Divide : Product  Inputs=*/
  Relational Operator : RelationalOperator  Operator===  OutDataTypeStr=boolean  RndMeth=Simplest
  Subtract : Sum  Inputs=+-
  "Available " : Outport
  Cnt : Outport  Port=2
  Timeout_Err : Outport  Port=3
  Msg_Freq : Outport  Port=4
  wires:
  Delay3/1 -> Subtract/1
  Constant/1 -> Divide/2
  Divide/1 -> Msg_Freq/1
  Data Type Conversion/1 -> Divide/1
  Delay2/1 -> Subtract/2
  Delay1/1 -> Relational Operator/2
  Msg_cnt/1 -> Cnt/1, Delay2/1, Delay1/1, Delay3/1, Relational Operator/1
  Relational Operator/1 -> Timeout_Err/1
  Subtract/1 -> Data Type Conversion/1
  "Available_in "/1 -> "Available "/1

== system Ecotron/Input/By-wire/Robeff Brake ECU/Robeff Brake FbMsg3/Subsystem4 ==
  "Available_in " : Inport
  Msg_cnt : Inport  Port=2
  Constant : Constant  Value=3  OutDataTypeStr=single
  Data Type Conversion : DataTypeConversion  OutDataTypeStr=single
  Delay1 : Delay  InitialCondition=0  SampleTime=0.5
  Delay2 : Delay  DelayLength=6  InitialCondition=0  SampleTime=0.5
  Delay3 : Delay  DelayLength=0  InitialCondition=0  SampleTime=0.5
  Divide : Product  Inputs=*/
  Relational Operator : RelationalOperator  Operator===  OutDataTypeStr=boolean  RndMeth=Simplest
  Subtract : Sum  Inputs=+-
  "Available " : Outport
  Cnt : Outport  Port=2
  Timeout_Err : Outport  Port=3
  Msg_Freq : Outport  Port=4
  wires:
  Delay3/1 -> Subtract/1
  Constant/1 -> Divide/2
  Divide/1 -> Msg_Freq/1
  Data Type Conversion/1 -> Divide/1
  Delay2/1 -> Subtract/2
  Delay1/1 -> Relational Operator/2
  Msg_cnt/1 -> Cnt/1, Delay2/1, Delay1/1, Delay3/1, Relational Operator/1
  Relational Operator/1 -> Timeout_Err/1
  Subtract/1 -> Data Type Conversion/1
  "Available_in "/1 -> "Available "/1

== system Ecotron/Input/By-wire/Robeff EPAS ECU/Robeff EPAS FbMsg1/Subsystem4 ==
  "Available_in " : Inport
  Msg_cnt : Inport  Port=2
  Constant : Constant  Value=3
  Data Type Conversion : DataTypeConversion  OutDataTypeStr=single
  Delay1 : Delay  InitialCondition=0  SampleTime=0.5
  Delay2 : Delay  DelayLength=6  InitialCondition=0  SampleTime=0.5
  Delay3 : Delay  DelayLength=0  InitialCondition=0  SampleTime=0.5
  Divide : Product  Inputs=*/  OutDataTypeStr=single
  Relational Operator : RelationalOperator  Operator===  OutDataTypeStr=boolean  RndMeth=Simplest
  Subtract : Sum  Inputs=+-
  "Available " : Outport
  Cnt : Outport  Port=2
  Timeout_Err : Outport  Port=3
  Msg_Freq : Outport  Port=4
  wires:
  "Available_in "/1 -> "Available "/1
  Subtract/1 -> Data Type Conversion/1
  Relational Operator/1 -> Timeout_Err/1
  Msg_cnt/1 -> Relational Operator/1, Delay3/1, Delay1/1, Delay2/1, Cnt/1
  Delay1/1 -> Relational Operator/2
  Delay2/1 -> Subtract/2
  Data Type Conversion/1 -> Divide/1
  Divide/1 -> Msg_Freq/1
  Constant/1 -> Divide/2
  Delay3/1 -> Subtract/1

== system Ecotron/Input/By-wire/Robeff EPAS ECU/Robeff EPAS FbMsg2/Subsystem4 ==
  "Available_in " : Inport
  Msg_cnt : Inport  Port=2
  Constant : Constant  Value=3
  Data Type Conversion : DataTypeConversion  OutDataTypeStr=single
  Delay1 : Delay  InitialCondition=0  SampleTime=0.5
  Delay2 : Delay  DelayLength=6  InitialCondition=0  SampleTime=0.5
  Delay3 : Delay  DelayLength=0  InitialCondition=0  SampleTime=0.5
  Divide : Product  Inputs=*/  OutDataTypeStr=single
  Relational Operator : RelationalOperator  Operator===  OutDataTypeStr=boolean  RndMeth=Simplest
  Subtract : Sum  Inputs=+-
  "Available " : Outport
  Cnt : Outport  Port=2
  Timeout_Err : Outport  Port=3
  Msg_Freq : Outport  Port=4
  wires:
  "Available_in "/1 -> "Available "/1
  Subtract/1 -> Data Type Conversion/1
  Relational Operator/1 -> Timeout_Err/1
  Msg_cnt/1 -> Relational Operator/1, Delay3/1, Delay1/1, Delay2/1, Cnt/1
  Delay1/1 -> Relational Operator/2
  Delay2/1 -> Subtract/2
  Data Type Conversion/1 -> Divide/1
  Divide/1 -> Msg_Freq/1
  Constant/1 -> Divide/2
  Delay3/1 -> Subtract/1

== system Ecotron/Input/By-wire/Robeff EPAS ECU/Robeff EPAS FbMsg3/Subsystem4 ==
  "Available_in " : Inport
  Msg_cnt : Inport  Port=2
  Constant : Constant  Value=3
  Data Type Conversion : DataTypeConversion  OutDataTypeStr=single
  Delay1 : Delay  InitialCondition=0  SampleTime=0.5
  Delay2 : Delay  DelayLength=6  InitialCondition=0  SampleTime=0.5
  Delay3 : Delay  DelayLength=0  InitialCondition=0  SampleTime=0.5
  Divide : Product  Inputs=*/  OutDataTypeStr=single
  Relational Operator : RelationalOperator  Operator===  OutDataTypeStr=boolean  RndMeth=Simplest
  Subtract : Sum  Inputs=+-
  "Available " : Outport
  Cnt : Outport  Port=2
  Timeout_Err : Outport  Port=3
  Msg_Freq : Outport  Port=4
  wires:
  "Available_in "/1 -> "Available "/1
  Subtract/1 -> Data Type Conversion/1
  Relational Operator/1 -> Timeout_Err/1
  Msg_cnt/1 -> Relational Operator/1, Delay3/1, Delay1/1, Delay2/1, Cnt/1
  Delay1/1 -> Relational Operator/2
  Delay2/1 -> Subtract/2
  Data Type Conversion/1 -> Divide/1
  Divide/1 -> Msg_Freq/1
  Constant/1 -> Divide/2
  Delay3/1 -> Subtract/1

== system Ecotron/Main /LongControl /ACC Control/Fcalculator /Acceleration1 ==
  speed : Inport
  Moving Average1 : dspstat3/Moving Average  Method=Sliding window  ForgettingFactorPort=off  SpecifyWindowLength=on  WindowLength=200  ForgettingFactor=0.9  SimulateUsing=Code generation
  Moving Average2 : dspstat3/Moving Average  Method=Sliding window  ForgettingFactorPort=off  SpecifyWindowLength=on  WindowLength=200  ForgettingFactor=0.9  SimulateUsing=Code generation
  basic derivative1 : Subsystem
  m/s^2 : Outport
  wires:
  Moving Average2/1 -> m/s^2/1  "m/s^2"
  basic derivative1/1(Out1) -> Moving Average2/1
  speed/1 -> Moving Average1/1
  Moving Average1/1 -> basic derivative1/1(In1)  "m/s"

== system Ecotron/Main /LongControl /ACC Control/Fcalculator /Gearbox loss ==
  Constant : Constant  Value=1.06
  Out1 : Outport
  wires:
  Constant/1 -> Out1/1

== system Ecotron/Main /LongControl /ACC Control/Fcalculator /Rolling resistance ==
  In1 : Inport
  1-D Lookup Table : Lookup_n-D  NumberOfTableDimensions=1  BreakpointsForDimension1=[0 0.02 8 16]  Table=[0 163.2 228.5 326.4]  InternalRulePriority=Speed  RndMeth=Simplest  InputSameDT=on
  Out1 : Outport
  wires:
  1-D Lookup Table/1 -> Out1/1
  In1/1 -> 1-D Lookup Table/1

== system Ecotron/Main /LongControl /ACC Control/Fcalculator /Subsystem ==
  In1 : Inport
  <GOLF_MotorTorque> : Inport  Port=2
  reset : Inport  Port=3
  PID Controller1 : simulink/Continuous/PID Controller  Controller=PID  Form=Parallel  TimeDomain=Discrete-time  SampleTime=1/100  IntegratorMethod=Forward Euler  FilterMethod=Forward Euler  ControllerParametersSource=external  P=1  I=1  D=0  UseFilter=off  N=100  TunerSelectOption=Transfer Function Based (PID Tuner App)  ZeroCross=off  InitialConditionSource=internal  InitialConditionForIntegrator=0  InitialConditionForFilter=0  DifferentiatorICPrevScaledInput=0  ExternalReset=either  TrackingMode=off  Kt=1  LimitOutput=on  UpperSaturationLimit=50  LowerSaturationLimit=0  LinearizeAsGain=off  AntiWindupMode=clamping  Kb=1  POutMin=[]  POutMax=[]  IOutMin=[]  IOutMax=[]  DOutMin=[]  DOutMax=[]  NOutMin=[]  NOutMax=[]  SumOutMin=[]  SumOutMax=[]  SaturationOutMin=[]  SaturationOutMax=[]  PParamMin=[]  PParamMax=[]  IParamMin=[]  IParamMax=[]  DParamMin=[]  DParamMax=[]  NParamMin=[]  NParamMax=[]  KbParamMin=[]  KbParamMax=[]  KtParamMin=[]  KtParamMax=[]  KbOutMin=[]  KbOutMax=[]  KtOutMin=[]  KtOutMax=[]  IntegratorOutMin=[]  IntegratorOutMax=[]  FilterOutMin=[]  FilterOutMax=[]  SumI1OutMin=[]  SumI1OutMax=[]  SumI2OutMin=[]  SumI2OutMax=[]  SumI3OutMin=[]  SumI3OutMax=[]  SumI4OutMin=[]  SumI4OutMax=[]  SumDOutMin=[]  SumDOutMax=[]  DifferentiatorOutMin=[]  DifferentiatorOutMax=[]  FilterDiffOutCoefMin=[]  FilterDiffOutCoefMax=[]  ReciprocalOutMin=[]  ReciprocalOutMax=[]  SumDenOutMin=[]  SumDenOutMax=[]  SumNumOutMin=[]  SumNumOutMax=[]  DivideOutMin=[]  DivideOutMax=[]  IntegratorContinuousStateAttributes=''  IntegratorStateMustResolveToSignalObject=off  IntegratorRTWStateStorageClass=Auto  FilterContinuousStateAttributes=''  FilterStateMustResolveToSignalObject=off  FilterRTWStateStorageClass=Auto  ParallelPVariant=ExternalParameters  IdealPVariant=Disabled  IVariant=ExternalParameters  DVariant=ExternalParameters  IntegratorVariant=Discrete  SatVariant=Enabled  AWVariant=DiscClampingParallel  PCopyVariant=Disabled  TRVariant=Disabled  FdbkBlocksVariant=Forward  IdealPFdbkVariant=Disabled  SatFdbkVariant=Disabled  DerivativeFilterVariant=Differentiator  NVariant=Passthrough  NCopyVariant=Disabled_SignalSpec  FilterICVariant=InternalICsDifferentiator  IntegratorICVariant=InternalICs  ExternalResetVariant=ExternalReset  TRSumVariant=Passthrough  SumFdbkVariant=Disabled  SumVariant=Sum_PID
  Read Calibration : CoderSF_BSW_Libs/Calibration & Measurement/Read Calibration  variable_name=Torque_PID_P  variable_value=0.05  variable_type=single  variable_min=[]  variable_max=[]  unitStr=""  descStr=""
      settings: AttributesFormatString=value:%<variable_value> type:%<variable_type> max:%<variable_max> Min:%<variable_min>  SourceProductName=EcoCoder Blocks
  Read Calibration1 : CoderSF_BSW_Libs/Calibration & Measurement/Read Calibration  variable_name=Torque_PID_I  variable_value=0.3  variable_type=single  variable_min=[]  variable_max=[]  unitStr=""  descStr=""
      settings: AttributesFormatString=value:%<variable_value> type:%<variable_type> max:%<variable_max> Min:%<variable_min>  SourceProductName=EcoCoder Blocks
  Read Calibration2 : CoderSF_BSW_Libs/Calibration & Measurement/Read Calibration  variable_name=Torque_PID_D  variable_value=0  variable_type=single  variable_min=[]  variable_max=[]  unitStr=""  descStr=""
      settings: AttributesFormatString=value:%<variable_value> type:%<variable_type> max:%<variable_max> Min:%<variable_min>  SourceProductName=EcoCoder Blocks
  Subtract1 : Sum  Inputs=+-
  Out1 : Outport
  wires:
  Subtract1/1 -> PID Controller1/1
  Read Calibration2/1 -> PID Controller1/4
  Read Calibration/1 -> PID Controller1/2
  Read Calibration1/1 -> PID Controller1/3
  PID Controller1/1 -> Out1/1
  In1/1 -> Subtract1/1
  <GOLF_MotorTorque>/1 -> Subtract1/2
  reset/1 -> PID Controller1/5

== system Ecotron/Main /LongControl /ACC Control/Fcalculator /Subsystem1 ==
  In1 : Inport
  <Brake pressure> : Inport  Port=2
  reset : Inport  Port=3
  PID Controller1 : simulink/Continuous/PID Controller  Controller=PID  Form=Parallel  TimeDomain=Discrete-time  SampleTime=1/100  IntegratorMethod=Forward Euler  FilterMethod=Forward Euler  ControllerParametersSource=external  P=1  I=1  D=0  UseFilter=off  N=100  TunerSelectOption=Transfer Function Based (PID Tuner App)  ZeroCross=off  InitialConditionSource=internal  InitialConditionForIntegrator=10  InitialConditionForFilter=0  DifferentiatorICPrevScaledInput=0  ExternalReset=either  TrackingMode=off  Kt=1  LimitOutput=on  UpperSaturationLimit=120  LowerSaturationLimit=0  LinearizeAsGain=off  AntiWindupMode=clamping  Kb=1  POutMin=[]  POutMax=[]  IOutMin=[]  IOutMax=[]  DOutMin=[]  DOutMax=[]  NOutMin=[]  NOutMax=[]  SumOutMin=[]  SumOutMax=[]  SaturationOutMin=[]  SaturationOutMax=[]  PParamMin=[]  PParamMax=[]  IParamMin=[]  IParamMax=[]  DParamMin=[]  DParamMax=[]  NParamMin=[]  NParamMax=[]  KbParamMin=[]  KbParamMax=[]  KtParamMin=[]  KtParamMax=[]  KbOutMin=[]  KbOutMax=[]  KtOutMin=[]  KtOutMax=[]  IntegratorOutMin=[]  IntegratorOutMax=[]  FilterOutMin=[]  FilterOutMax=[]  SumI1OutMin=[]  SumI1OutMax=[]  SumI2OutMin=[]  SumI2OutMax=[]  SumI3OutMin=[]  SumI3OutMax=[]  SumI4OutMin=[]  SumI4OutMax=[]  SumDOutMin=[]  SumDOutMax=[]  DifferentiatorOutMin=[]  DifferentiatorOutMax=[]  FilterDiffOutCoefMin=[]  FilterDiffOutCoefMax=[]  ReciprocalOutMin=[]  ReciprocalOutMax=[]  SumDenOutMin=[]  SumDenOutMax=[]  SumNumOutMin=[]  SumNumOutMax=[]  DivideOutMin=[]  DivideOutMax=[]  IntegratorContinuousStateAttributes=''  IntegratorStateMustResolveToSignalObject=off  IntegratorRTWStateStorageClass=Auto  FilterContinuousStateAttributes=''  FilterStateMustResolveToSignalObject=off  FilterRTWStateStorageClass=Auto  ParallelPVariant=ExternalParameters  IdealPVariant=Disabled  IVariant=ExternalParameters  DVariant=ExternalParameters  IntegratorVariant=Discrete  SatVariant=Enabled  AWVariant=DiscClampingParallel  PCopyVariant=Disabled  TRVariant=Disabled  FdbkBlocksVariant=Forward  IdealPFdbkVariant=Disabled  SatFdbkVariant=Disabled  DerivativeFilterVariant=Differentiator  NVariant=Passthrough  NCopyVariant=Disabled_SignalSpec  FilterICVariant=InternalICsDifferentiator  IntegratorICVariant=InternalICs  ExternalResetVariant=ExternalReset  TRSumVariant=Passthrough  SumFdbkVariant=Disabled  SumVariant=Sum_PID
  Read Calibration : CoderSF_BSW_Libs/Calibration & Measurement/Read Calibration  variable_name=Brake_PID_P  variable_value=3  variable_type=single  variable_min=[]  variable_max=[]  unitStr=""  descStr=""
      settings: AttributesFormatString=value:%<variable_value> type:%<variable_type> max:%<variable_max> Min:%<variable_min>  SourceProductName=EcoCoder Blocks
  Read Calibration1 : CoderSF_BSW_Libs/Calibration & Measurement/Read Calibration  variable_name=Brake_PID_I  variable_value=5  variable_type=single  variable_min=[]  variable_max=[]  unitStr=""  descStr=""
      settings: AttributesFormatString=value:%<variable_value> type:%<variable_type> max:%<variable_max> Min:%<variable_min>  SourceProductName=EcoCoder Blocks
  Read Calibration2 : CoderSF_BSW_Libs/Calibration & Measurement/Read Calibration  variable_name=Brake_PID_D  variable_value=0  variable_type=single  variable_min=[]  variable_max=[]  unitStr=""  descStr=""
      settings: AttributesFormatString=value:%<variable_value> type:%<variable_type> max:%<variable_max> Min:%<variable_min>  SourceProductName=EcoCoder Blocks
  Subtract1 : Sum  Inputs=+-
  Out1 : Outport
  wires:
  <Brake pressure>/1 -> Subtract1/2
  In1/1 -> Subtract1/1
  PID Controller1/1 -> Out1/1
  Read Calibration1/1 -> PID Controller1/3
  Read Calibration/1 -> PID Controller1/2
  Read Calibration2/1 -> PID Controller1/4
  Subtract1/1 -> PID Controller1/1
  reset/1 -> PID Controller1/5

== system Ecotron/Main /LongControl /ACC Control/Fcalculator /motorbrake ==
  motor torque : Inport
  Gear : Inport  Port=2
  1-D Lookup Table : Lookup_n-D  NumberOfTableDimensions=1  BreakpointsForDimension1=[0 1 2 3 4 5]  Table=[0 53.5 32.6 21.7 16.2 12.2]  InternalRulePriority=Speed  RndMeth=Simplest  InputSameDT=on
  Product : Product
  Saturation : Saturate  UpperLimit=0  LowerLimit=-inf
  Out1 : Outport
  wires:
  Gear/1 -> 1-D Lookup Table/1
  1-D Lookup Table/1 -> Product/2
  motor torque/1 -> Product/1
  Product/1 -> Saturation/1
  Saturation/1 -> Out1/1

== system Ecotron/Main /LongControl /ACC Control/Fcalculator /slope ==
  kg : Inport
  pitch : Inport  Port=2
  Constant : Constant  Value=9.81
  Gain : Gain  Gain=0.01
  Product : Product  Inputs=3
  Out1 : Outport
  wires:
  kg/1 -> Product/1
  pitch/1 -> Gain/1
  Constant/1 -> Product/3
  Product/1 -> Out1/1
  Gain/1 -> Product/2
